simulink model "raised_cosine_3"  (Simulink 5.0)
settings: Solver=ode45  StartTime=0.0  StopTime=10.0  RelTol=1e-3
values from neighbouring files (symbols this model uses):
  nord = 6    [analog_bp1.m]    (also in analog_bp2.m; analog_bp3.m; analog_tp1.m = 8; analog_tp2.m = 8)
  Ts = 1/fs    (= 6.25e-05)    [G722_1.m]    (also in adaptiv_2.m = 0.001; adaptiv_3.m = 0.001; adaptiv_4.m = 0.001; adaptiv_5.m = 0.001)
undefined symbols (not defined in the file or in its folder): Fs, get, hrc_puls, Tsymb
libraries: dspsigops x3, dspbuff3 x2, dspspect3 x2, dspstat3 x2, simulink x1, dspsnks4 x1
settings Model: Creator=svenhoffmann  LastModifiedBy=svenhoffmann  ExtModeAutoUpdateStatusClock=off  MaxDataPoints=5000

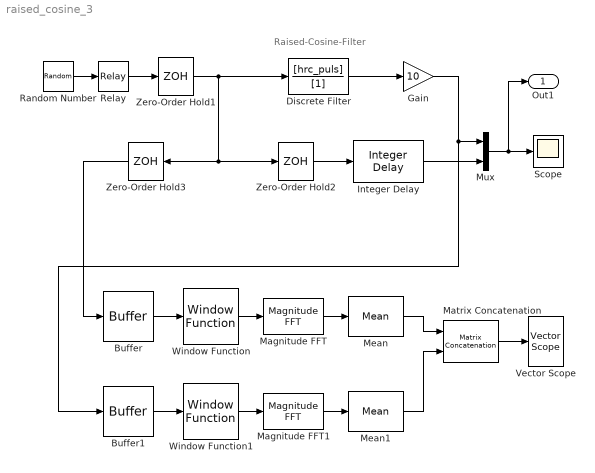
== system raised_cosine_3 ==
  note: Raised-Cosine-Filter
  Buffer : dspbuff3/Buffer  N=256  V=0  ic=0
  Buffer1 : dspbuff3/Buffer  N=256  V=0  ic=0
  Discrete Filter : DiscreteFilter  Numerator=[hrc_puls]  Denominator=[1]  SampleTime=Ts
  Gain : Gain  Gain=10  SaturateOnIntegerOverflow=on
  Integer Delay : dspsigops/Integer Delay  delay=nord/2  ic=0  reset_popup=None
  Magnitude FFT : dspspect3/Magnitude FFT  mag_or_magsq=Magnitude squared  fftLenInherit=off  fftsize=256
  Magnitude FFT1 : dspspect3/Magnitude FFT  mag_or_magsq=Magnitude squared  fftLenInherit=off  fftsize=256
  Matrix Concatenation : simulink/Math Operations/Matrix Concatenation  numInports=2  catMethod=Horizontal
  Mean : dspstat3/Mean  run=on  reset_popup=None
  Mean1 : dspstat3/Mean  run=on  reset_popup=None
  Mux : Mux  Inputs=2
  Random Number : RandomNumber  SampleTime=0
  Relay : Relay  OffOutputValue=-1
  Scope : Scope
  Vector Scope : dspsnks4/Vector Scope  ScopeProperties=off  Domain=Frequency  HorizSpan=1  DisplayProperties=off  AxisGrid=on  Memory=off  FrameNumber=on  AxisLegend=off  AxisZoom=off  OpenScopeAtSimStart=on  OpenScopeImmediately=off  FigPos=get(0,'defaultfigureposition')  AxisProperties=on  XUnits=Hertz  XRange=[-Fs/2...Fs/2]  InheritXIncr=off  XIncr=Ts  XLabel=Time  YUnits=dB  YLabel=Amplitude  LineProperties=off
      settings: YMin=-27.3525697963528  YMax=34.9252389184608
  Window Function : dspsigops/Window Function  winmode=Apply window to input  wintype=Hamming  N=64  Rs=50  beta=10  winsamp=Symmetric  UserWindow=hamming  OptParams=off  UserParams={1.0}  datatype=Double
  Window Function1 : dspsigops/Window Function  winmode=Apply window to input  wintype=Hamming  N=64  Rs=50  beta=10  winsamp=Symmetric  UserWindow=hamming  OptParams=off  UserParams={1.0}  datatype=Double
  Zero-Order Hold1 : ZeroOrderHold  SampleTime=Tsymb
  Zero-Order Hold2 : ZeroOrderHold  SampleTime=Ts
  Zero-Order Hold3 : ZeroOrderHold  Orientation=left  SampleTime=Ts
  Out1 : Outport
  wires:
  Random Number/1 -> Relay/1
  Relay/1 -> Zero-Order Hold1/1
  Zero-Order Hold1/1 -> Zero-Order Hold2/1, Zero-Order Hold3/1, Discrete Filter/1
  Integer Delay/1 -> Mux/2
  Mux/1 -> Scope/1, Out1/1
  Discrete Filter/1 -> Gain/1
  Zero-Order Hold2/1 -> Integer Delay/1
  Gain/1 -> Buffer1/1, Mux/1
  Zero-Order Hold3/1 -> Buffer/1
  Buffer/1 -> Window Function/1
  Buffer1/1 -> Window Function1/1
  Magnitude FFT/1 -> Mean/1
  Magnitude FFT1/1 -> Mean1/1
  Matrix Concatenation/1 -> Vector Scope/1
  Window Function/1 -> Magnitude FFT/1
  Window Function1/1 -> Magnitude FFT1/1
  Mean/1 -> Matrix Concatenation/1
  Mean1/1 -> Matrix Concatenation/2
